simulink model "VirtualMotoTemplate"  (R2025b)
settings: Solver=daessc  StartTime=0  StopTime=2474  FixedStep=.001  RelTol=1e-2  EnableMultiTasking=on
StopFcn:
  | %toc
undefined symbols (not defined in the file): AccelOvrCmd, CtrlTcuInitGear, DecelOvrCmd, Disabled, DriverPreviewDist, EnblAccelOvr, EnblDecelCmd, EnblSteerCmd, EnvAbsPrs, EnvAirTemp, EnvGrvty, EnvNomFrictionScaling, EnvNominalGrade, EnvWindVelX, EnvWindVelY, EnvWindVelZ, FTP75, MotoFrmInert, MotoFrmLngth, MotoFrmMass, MotoLowrFrntFrkMass, MotoRearArmLngth, MotoRearArmMass, MotoUpprFrntFrkMass, RiderLkAhdPtDstGain, RiderMass, ScnAccTbl, ScnBrkTbl, ScnCRMaxLatAccel, ScnCRRadius, ScnDLCGateLongPos, ScnDLCLatRef, ScnDLCLatRefOffset, ScnDLCLongRefBpt, ScnDLCLongRefStartPos, ScnDLCVehicleWidth, ScnFHCounterDwellTime, ScnFHInitialDwellTime, ScnFHReturnTime, ScnFHRollRateZeroCross, ScnFHSteerAmp, ScnFHSteerSpeed, ScnISHandwheelRate, ScnISMaxHandwheelAng, ScnISMaxLatAccel, ScnISSteerHoldTime, ScnLongPosBpts, ScnLongVelRef, ScnOvalTrackl, ScnOvalTrackpdst, ScnOvalTrackr, ScnSDDwellTime, ScnSDSteerAmp, ScnSDSteerFreq, ScnSSFinalFreq, ScnSSSteerAmp, ScnSSSweepTime, ScnStartTime, ScnStrgAngTbl, ScnStrgTrqTbl ... (+10)
libraries: simulink x16, vehdynlibscenariocommon x9, sm_lib x6, autolibshared x4, nesl_utility x4, vehdynlibviscommon x3, sim3dgroundtruthsensorlib x2, vehdynlibdriver x2, sharedtransform x1, autolibutils x1, sim3dautolib x1, sim3dlib x1
(part 5 of 6)

== system VirtualMotoTemplate/Rider Commands/Rider Commands/Roll angle control/Rider Steering Control ==
  sensors : Inport
  TargetRollAngle : Inport  Port=2
  Bus Selector1 : BusSelector  OutputSignals=Wheels.RearTire.Vx,Wheels.RearTire.Gamma,Wheels.RearTire.phidot,Wheels.RearTire.X,Wheels.RearTire.Y,Body.InertFrm.Cg.Ang.psi
  Rider Steering : Subsystem  Variant=on  VariantControlMode=label  VariantControl=Choice  LabelModeActiveChoice=Roll angle control  mask{RiderControlTypePanel=Roll angle control, TrajectoryTypePanel=Oval, RidTrajContG=RidTrajContG, RidTrajContGphi=RidTrajContGphi, RidTrajContGphid=RidTrajContGphid, RidTrajContGl=RidTrajContGl, RidTrajContTD=RidTrajContTD, RidTrajContTL=RidTrajContTL, RidRollContGphi=RidRollContGphi, RidRollContGphid=RidRollContGphid, Trajr=Trajr, Trajl=Trajl, Trajpointdist=Trajpointdist, TrajDatFile=TrajDatFile}
      mask prompts: RiderControlTypePanel "Rider control type:"; TrajectoryTypePanel "Trajectory type:"; RidTrajContG "Gain to determine the Target roll angle, RidContG [rad/m]:"; RidTrajContGphi "Gain to follow the Target trajectory, RidContGphi [Nm/rad]:"; RidTrajContGphid "Gain to prevent the vehicle from tipping over, RidContGphid [Nms/rad]:"; RidTrajContGl "Gain that determines the distance to the look ahead point, RidContGl [s]:"; RidTrajContTD "Time constant for 1st order delay, RidContTD [s]:"; RidTrajContTL "Dead time of rider operation, RidContTL [s]:"; RidRollContGphi "Gain to follow the Target trajectory, RidContGphi [Nm/rad]:"; RidRollContGphid "Gain to prevent the vehicle from tipping over, RidContGphid [Nms/rad]:"; Trajr "Trajectory parameter,Trajr [m]:"; Trajl "Trajectory parameter,Trajl [m]:"; Trajpointdist ",Trajpdist [m]:"; TrajDatFile "Trajectory data file:"
      mask init:
      | maskObj = Simulink.Mask.get(gcb);
      | 
      | Type_tmp = maskObj.getParameter('TrajectoryTypePanel');
      | Type     = Type_tmp.Value;
      | 
      | switch Type
      |     case 'Oval'
      | % ------------------------------------------------------------------------%
      | %  Create Trajectory
      | % ------------------------------------------------------------------------%
      | % --- Oval --- %
      | % top part %
      | x_straight1 = -Trajl/2:Trajpointdist:Trajl/2;
      | y_straight1 = x_straight1*0;
      | 
      | % bottom part %
      | x_straight2 = -Trajl/2:Trajpointdist:Trajl/2;
      | y_straight2 = x_straight1*0+2*Trajr;
      | 
      | % right part %
      | theta_corner1 = -pi/2:Trajpointdist/Trajr:pi/2;
      | x_corner1     = Trajr*cos(theta_corner1)+Trajl/2;
      | y_corner1     = Trajr*sin(theta_corner1)+Trajr;
      | 
      | % left part %
      | theta_corner2 = pi/2:Trajpointdist/Trajr:3/2*pi;
      | x_corner2     = Trajr*cos(theta_corner2)-Trajl/2;
      | y_corner2     = Trajr*sin(theta_corner2)+Trajr;
      | 
      | % total %
      | x_oval = [x_straight1, x_corner1(2:end), fliplr(x_straight2), x_corner2(2:end)];
      | y_oval = [y_straight1, y_corner1(2:end), fliplr(y_straight2), y_corner2(2:end)];
      | 
      | trackData(1,:) = x_oval;
      | trackData(2,:) = y_oval;
      | trackData(3,:) = y_oval*0;
      | 
      |     case 'User defined'
      | 
      | TmpTraj = load(TrajDatFile);
      | 
      | trackData(1,:) = TmpTraj.TrajX;
      | trackData(2,:) = -TmpTraj.TrajY;
      | trackData(3,:) = TmpTraj.TrajY*0;
      | 
      | end
      mask Callback RiderControlTypePanel:
      | maskObj = Simulink.Mask.get(gcb);
      | 
      | Type_tmp = maskObj.getParameter('RiderControlTypePanel');
      | Type     = Type_tmp.Value;
      | 
      | TrajGroup = maskObj.getDialogControl('RiderTrajectoryControlParamPanel');
      | RollGroup = maskObj.getDialogControl('RiderRollControlParamPanel');
      | 
      | TrajectoryTypePanel = maskObj.getDialogControl('TrajectoryTypeCont');
      | TargetTrajectoryParamGroup = maskObj.getDialogControl('TargetTrajectoryParamGroup');
      | 
      | GroupAll = maskObj.getDialogControl('RiderControlParamGroup');
      | 
      | switch Type
      |     case 'None'
      |     set_param(gcb,'LabelModeActiveChoice', 'None');
      |     TrajGroup.Visible = 'off';
      |     RollGroup.Visible = 'off';
      |     GroupAll.Visible  = 'off';
      |     TrajectoryTypePanel.Visible = 'off';
      |     TargetTrajectoryParamGroup.Visible = 'off';
      |     case 'Target trajectory driving - Look ahead point'
      |     set_param(gcb,'LabelModeActiveChoice', 'Target trajectory driving - Look ahead point');
      |     TrajGroup.Visible = 'on';
      |     RollGroup.Visible = 'off';
      |     GroupAll.Visible  = 'on';
      |     TrajectoryTypePanel.Visible = 'on';
      |     TargetTrajectoryParamGroup.Visible = 'on';
      |     case 'Roll angle control'
      |     set_param(gcb,'LabelModeActiveChoice','Roll angle control');
      |     TrajGroup.Visible = 'off';
      |     RollGroup.Visible = 'on';
      |     GroupAll.Visible  = 'on';
      |     TrajectoryTypePanel.Visible = 'off';
      |     TargetTrajectoryParamGroup.Visible = 'off';
      |     case 'External'
      |     set_param(gcb,'LabelModeActiveChoice', 'External');
      |     TrajGroup.Visible = 'off';
      |     RollGroup.Visible = 'off';
      |     GroupAll.Visible  = 'off';
      |     TrajectoryTypePanel.Visible = 'off';
      |     TargetTrajectoryParamGroup.Visible = 'off';
      | end
      mask TypeOptions TrajectoryTypePanel: Oval | User defined
      mask Callback TrajectoryTypePanel:
      | maskObj = Simulink.Mask.get(gcb);
      | 
      | Type_tmp = maskObj.getParameter('TrajectoryTypePanel');
      | Type     = Type_tmp.Value;
      | 
      | TargetTrajectoryParamOvalPanel = maskObj.getDialogControl('TargetTrajectoryParamOvalPanel');
      | 
      | TargetTrajectoryParamUserDefinedPanel = maskObj.getDialogControl('TargetTrajectoryParamUserDefinedPanel');
      | 
      | TargetTrajectoryParamGroup = maskObj.getDialogControl('TargetTrajectoryParamGroup');
      | 
      | switch Type
      |     case 'Oval'
      | TargetTrajectoryParamGroup.Visible = 'on';
      | TargetTrajectoryParamOvalPanel.Visible        = 'on';
      | TargetTrajectoryParamUserDefinedPanel.Visible = 'off';
      |     case 'User defined'
      | TargetTrajectoryParamGroup.Visible = 'on';
      | TargetTrajectoryParamOvalPanel.Visible        = 'off';
      | TargetTrajectoryParamUserDefinedPanel.Visible = 'on';
      | end
      mask DialogControl RiderOptionsGroup Prompt: Options
      mask DialogControl RiderTrajectoryControlParamPanel Prompt: Control parameters
      mask DialogControl RiderRollControlParamPanel Prompt: Control parameters
      mask DialogControl TargetTrajectoryParamOvalPanel Prompt: Trajectory parameters
      mask DialogControl OvalTrajConfBtn Prompt: Confirm
      mask DialogControl OvalTrajConfBtn Callback:
      | maskObj = Simulink.Mask.get(gcb);
      | 
      | Trajr_tmp          = maskObj.getParameter('Trajr');
      | Trajr              = str2num(Trajr_tmp.Value);
      | Trajl_tmp          = maskObj.getParameter('Trajl');
      | Trajl              = str2num(Trajl_tmp.Value);
      | Trajpointdist_tmp  = maskObj.getParameter('Trajpointdist');
      | Trajpointdist      = str2num(Trajpointdist_tmp.Value);
      | 
      | % ------------------------------------------------------------------------%
      | %  Create Trajectory
      | % ------------------------------------------------------------------------%
      | % --- Oval --- %
      | % top part %
      | x_straight1 = -Trajl/2:Trajpointdist:Trajl/2;
      | y_straight1 = x_straight1*0;
      | 
      | % bottom part %
      | x_straight2 = -Trajl/2:Trajpointdist:Trajl/2;
      | y_straight2 = x_straight1*0+2*Trajr;
      | 
      | % right part %
      | theta_corner1 = -pi/2:Trajpointdist/Trajr:pi/2;
      | x_corner1     = Trajr*cos(theta_corner1)+Trajl/2;
      | y_corner1     = Trajr*sin(theta_corner1)+Trajr;
      | 
      | % left part %
      | theta_corner2 = pi/2:Trajpointdist/Trajr:3/2*pi;
      | x_corner2     = Trajr*cos(theta_corner2)-Trajl/2;
      | y_corner2     = Trajr*sin(theta_corner2)+Trajr;
      | 
      | % total %
      | x_oval = [x_straight1, x_corner1(2:end), fliplr(x_straight2), x_corner2(2:end)];
      | y_oval = [y_straight1, y_corner1(2:end), fliplr(y_straight2), y_corner2(2:end)];
      | 
      | figure;
      | plot(x_oval, -y_oval);
      | axis equal;
      | grid on;
      | xlabel('Coordinate X [m]');
      | ylabel('Coordinate Y [m]');
      | title('Oval target trajectory');
      | set(gca,'YDir','reverse')
      mask DialogControl TargetTrajectoryParamUserDefinedPanel Prompt: Trajectory parameters
      mask DialogControl UserDefinedTrajConfBtn Prompt: Confirm
      mask DialogControl UserDefinedTrajConfBtn Callback:
      | maskObj = Simulink.Mask.get(gcb);
      | 
      | File_tmp = maskObj.getParameter('TrajDatFile');
      | File     = replace(File_tmp.Value,'''','');
      | 
      | TmpTraj = load(File);
      | 
      | figure;
      | plot(TmpTraj.TrajX, TmpTraj.TrajY);
      | grid on;
      | xlabel('Coordinate X [m]');
      | ylabel('Coordinate Y [m]');
      | title('User defined target trajectory');
      | set(gca,'YDir','reverse');
  RiderInfo : Outport
  wires:
  sensors/1 -> Bus Selector1/1
  Rider Steering/1(Info) -> RiderInfo/1  "RiderInfo"
  TargetRollAngle/1 -> Rider Steering/7(Target roll angle)
  Bus Selector1/1 -> Rider Steering/1(dxdt)  "<Vx>"
  Bus Selector1/2 -> Rider Steering/2(roll)  "<Gamma>"
  Bus Selector1/3 -> Rider Steering/3(rollRate)  "<phidot>"
  Bus Selector1/4 -> Rider Steering/4(X)  "<X>"
  Bus Selector1/5 -> Rider Steering/5(Y)  "<Y>"
  Bus Selector1/6 -> Rider Steering/6(psi)  "<psi>"

== system VirtualMotoTemplate/Environment/Friction/Varying Friction/Road Track Friction/2D Lookup Tbl for Scaling Fctr (Lambda) ==
  XWhl : Inport  Partition=on  PartitionDimension=1  PartitionWidth=1  PartitionOffset=0
  YWhl : Inport  Port=2  Partition=on  PartitionDimension=1  PartitionWidth=1  PartitionOffset=0
  XBpt : Inport  Port=3
  YBpt : Inport  Port=4
  2-D Lookup Table : Lookup_n-D  BreakpointsForDimension1Source=Input port  BreakpointsForDimension1=xbr  BreakpointsForDimension2Source=Input port  BreakpointsForDimension2=ybr  Table=mutable  ExtrapMethod=Clip  InternalRulePriority=Speed  RndMeth=Simplest
      settings: InputPortMap=u0,u1,p5,p7
  For Each : ForEach  DisableCoverage=on
  Lambda for each whl : Outport  ConcatenationDimension=1
  wires:
  XWhl/1 -> 2-D Lookup Table/1
  YWhl/1 -> 2-D Lookup Table/2
  2-D Lookup Table/1 -> Lambda for each whl/1
  XBpt/1 -> 2-D Lookup Table/3
  YBpt/1 -> 2-D Lookup Table/4

== system VirtualMotoTemplate/Environment/Friction/Varying Friction/Road Track Friction/Creating Inertial Frm Bpt ==
  XCg : Inport
  YCg : Inport  Port=2
  Enable : EnablePort
  Add : Sum
  Add1 : Sum
  Constant1 : Constant  Value=ybr
  Constant3 : Constant  Value=xbr
  XBpt : Outport
  YBpt : Outport  Port=2
  wires:
  Add/1 -> XBpt/1
  Constant1/1 -> Add1/1
  Add1/1 -> YBpt/1
  Constant3/1 -> Add/2
  YCg/1 -> Add1/2
  XCg/1 -> Add/1

== system VirtualMotoTemplate/Environment/Friction/Varying Friction/Road Track Friction/En at t = 0 ==
  Clock1 : Clock
  Compare To Zero : simulink/Logic and Bit Operations/Compare To Zero  relop===  OutDataTypeStr=boolean
  Constant : Constant
  Constant2 : Constant  Value=0
  Switch1 : Switch  Criteria=u2 > Threshold  SaturateOnIntegerOverflow=off  InputSameDT=off
  Out1 : Outport
  wires:
  Clock1/1 -> Compare To Zero/1
  Constant2/1 -> Switch1/3
  Constant/1 -> Switch1/1
  Switch1/1 -> Out1/1
  Compare To Zero/1 -> Switch1/2

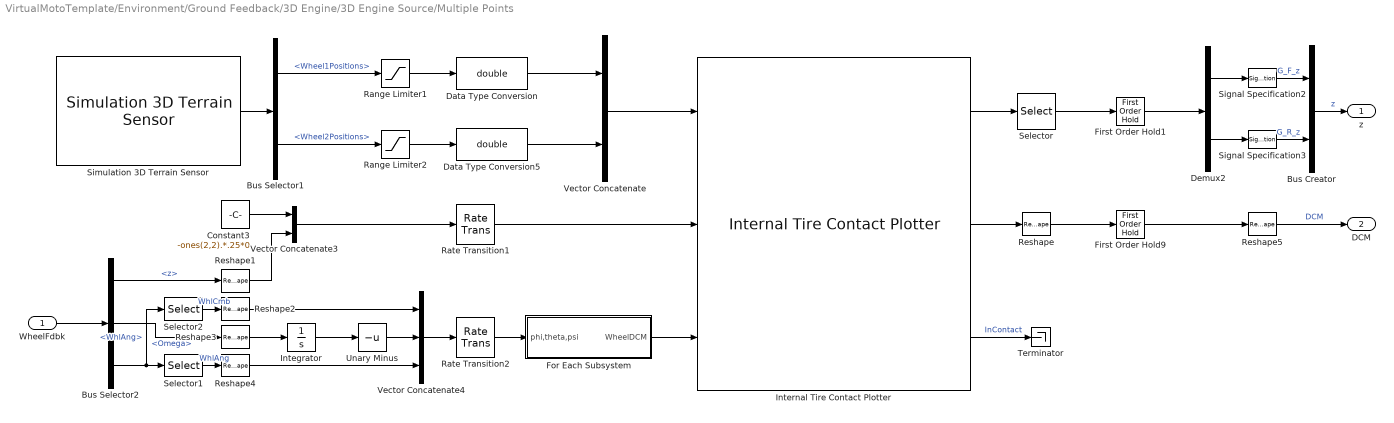
== system VirtualMotoTemplate/Environment/Ground Feedback/3D Engine/3D Engine Source/Multiple Points ==
  WheelFdbk : Inport
  Bus Creator : BusCreator  Inputs=2
  Bus Selector1 : BusSelector  OutputSignals=Wheel1Positions,Wheel2Positions
  Bus Selector2 : BusSelector  OutputSignals=z,Omega,WhlAng
  Constant3 : Constant  Value=-ones(2,2).*.25*0
  Data Type Conversion : DataTypeConversion  OutDataTypeStr=double  SaturateOnIntegerOverflow=off  RndMeth=Floor
  Data Type Conversion5 : DataTypeConversion  OutDataTypeStr=double  SaturateOnIntegerOverflow=off  RndMeth=Floor
  Demux2 : Demux  Outputs=2
  First Order Hold1 : FirstOrderHold  OutputAlgorithm=Fast (Minimize Error)  ErrorTolerance=.001
  First Order Hold9 : FirstOrderHold  InitialOutput=reshape(repmat(eye(3),1,1,2),[],1)  OutputAlgorithm=Fast (Minimize Error)  ErrorTolerance=.001
  For Each Subsystem : Subsystem  TreatAsAtomicUnit=on
  Integrator : Integrator  WrapState=on  ZeroCross=off
  Internal Tire Contact Plotter : vehdynlibviscommon/Internal Tire Contact Plotter  dispFig=off  numAxles=2  numWheelsPerAxle=1  wheelRad=.33  wheelWidth=.235  rayOrigins=[0.5 -0.5 0;0.4 -0.5 0;0.3 -0.5 0;0.19999999999999996 -0.5 0;0.099999999999999978 -0.5 0;0 -0.5 0;-0.099999999999999978 -0.5 0;-0.19999999999999996 -0.5 0;-0.3 -0.5 0;-0.4 -0.5 0;-0.5 -0.5 0;0.5 -0.4 0;0.4 -0.4 0;0.3 -0.4 0;0.19999999999999996 -0.4 0;0.099999999999999978 -0.4 0;0 -0.4 0;-0.099999999999999978 -0.4 0;-0.19999999999999996 -0.4 0;-0.3 -0.4 0;-0.4 -0.4 0;-0.5 -0.4 0;0.5 -0.3 0;0.4 -0.3 0;0.3 -0.3 0;0.19999999999999996 -0.3 0;0.099999999999999978 -0.3 0;0 -0.3 0;-0.099999999999999978 -0.3 0;-0.19999999999999996 -0.3 0;-0.3 -0.3 0;-0.4 -0.3 0;-0.5 -0.3 0;0.5 -0.19999999999999996 0;0.4 -0.19999999999999996 0;0.3 -0.19999999999999996 0;0.19999999999999996 -0.19999999999999996 0;0.099999999999999978 -0.19999999999999996 0;0 -0.19999999999999996 0;-0.099999999999999978 -0.19999999999999996 0;-0.19999999999999996 -0.19999999999999996 0;-0.3 -0.19999999999999996 0;-0.4 -0.19999999999999996 0;-0.5 -0.19999999999999996 0;0.5 -0.099999999999999978 0;0.4 -0.099999999999999978 0;0.3 -0.099999999999999978 0;0.19999999999999996 -0.099999999999999978 0;0.099999999999999978 -0.099999999999999978 0;0 -0.099999999999999978 0;-0.099999999999999978 -0.099999999999999978 0;-0.19999999999999996 -0.099999999999999978 0;-0.3 -0.099999999999999978 0;-0.4 -0.099999999999999978 0;-0.5 -0.099999999999999978 0;0.5 0 0;0.4 0 0;0.3 0 0;0.19999999999999996 0 0;0.099999999999999978 0 0;0 0 0;-0.099999999999999978 0 0;-0.19999999999999996 0 0;-0.3 0 0;-0.4 0 0;-0.5 0 0;0.5 0.099999999999999978 0;0.4 0.099999999999999978 0;0.3 0.099999999999999978 0;0.19999999999999996 0.099999999999999978 0;0.099999999999999978 0.099999999999999978 0;0 0.099999999999999978 0;-0.099999999999999978 0.099999999999999978 0;-0.19999999999999996 0.099999999999999978 0;-0.3 0.099999999999999978 0;-0.4 0.099999999999999978 0;-0.5 0.099999999999999978 0;0.5 0.19999999999999996 0;0.4 0.19999999999999996 0;0.3 0.19999999999999996 0;0.19999999999999996 0.19999999999999996 0;0.099999999999999978 0.19999999999999996 0;0 0.19999999999999996 0;-0.099999999999999978 0.19999999999999996 0;-0.19999999999999996 0.19999999999999996 0;-0.3 0.19999999999999996 0;-0.4 0.19999999999999996 0;-0.5 0.19999999999999996 0;0.5 0.3 0;0.4 0.3 0;0.3 0.3 0;0.19999999999999996 0.3 0;0.099999999999999978 0.3 0;0 0.3 0;-0.099999999999999978 0.3 0;-0.19999999999999996 0.3 0;-0.3 0.3 0;-0.4 0.3 0;-0.5 0.3 0;0.5 0.4 0;0.4 0.4 0;0.3 0.4 0;0.19999999999999996 0.4 0;0.099999999999999978 0.4 0;0 0.4 0;-0.099999999999999978 0.4 0;-0.19999999999999996 0.4 0;-0.3 0.4 0;-0.4 0.4 0;-0.5 0.4 0;0.5 0.5 0;0.4 0.5 0;0.3 0.5 0;0.19999999999999996 0.5 0;0.099999999999999978 0.5 0;0 0.5 0;-0.099999999999999978 0.5 0;-0.19999999999999996 0.5 0;-0.3 0.5 0;-0.4 0.5 0;-0.5 0.5 0]
  Range Limiter1 : Saturate  UpperLimit=1e3  LowerLimit=-1e3  ZeroCross=off
  Range Limiter2 : Saturate  UpperLimit=1e3  LowerLimit=-1e3  ZeroCross=off
  Rate Transition1 : RateTransition  Integrity=off  Deterministic=off  OutPortSampleTime=.01
  Rate Transition2 : RateTransition  Integrity=off  Deterministic=off  OutPortSampleTime=.01
  Reshape : Reshape  OutputDimensionality=Column vector (2-D)
  Reshape1 : Reshape  OutputDimensionality=Column vector (2-D)
  Reshape2 : Reshape  OutputDimensionality=Row vector (2-D)
  Reshape3 : Reshape  OutputDimensionality=Row vector (2-D)
  Reshape4 : Reshape  OutputDimensionality=Row vector (2-D)
  Reshape5 : Reshape  OutputDimensionality=Customize  OutputDimensions=[3,3,2]
  Selector : Selector  NumberOfDimensions=2  InputPortWidth=3  IndexOptions=Select all,Index vector (dialog)  Indices=[1 3],3  OutputSizes=1,1
  Selector1 : Selector  NumberOfDimensions=2  InputPortWidth=3  IndexOptions=Index vector (dialog),Select all  Indices=[3],1  OutputSizes=1,1
  Selector2 : Selector  NumberOfDimensions=2  InputPortWidth=3  IndexOptions=Index vector (dialog),Select all  Indices=[1],1  OutputSizes=1,1
  Signal Specification2 : SignalSpecification  Unit=m
  Signal Specification3 : SignalSpecification  Unit=m
  Simulation 3D Terrain Sensor : sim3dgroundtruthsensorlib/Simulation 3D Terrain Sensor  Priority=1  vehTagList={'Scene Origin';'SimulinkVehicle1'}  sensorTag=Sim3dSensor�  sensorId=1  sensorName=Sim3dSensor�  vehTag=SimulinkVehicle1  CoordinateSystem=Default  tmountOffset=[0, 0, 0]  rmountOffset=[0,0,0,]  RayOrigins=[0.5 -0.5 0;0.4 -0.5 0;0.3 -0.5 0;0.19999999999999996 -0.5 0;0.099999999999999978 -0.5 0;0 -0.5 0;-0.099999999999999978 -0.5 0;-0.19999999999999996 -0.5 0;-0.3 -0.5 0;-0.4 -0.5 0;-0.5 -0.5 0;0.5 -0.4 0;0.4 -0.4 0;0.3 -0.4 0;0.19999999999999996 -0.4 0;0.099999999999999978 -0.4 0;0 -0.4 0;-0.099999999999999978 -0.4 0;-0.19999999999999996 -0.4 0;-0.3 -0.4 0;-0.4 -0.4 0;-0.5 -0.4 0;0.5 -0.3 0;0.4 -0.3 0;0.3 -0.3 0;0.19999999999999996 -0.3 0;0.099999999999999978 -0.3 0;0 -0.3 0;-0.099999999999999978 -0.3 0;-0.19999999999999996 -0.3 0;-0.3 -0.3 0;-0.4 -0.3 0;-0.5 -0.3 0;0.5 -0.19999999999999996 0;0.4 -0.19999999999999996 0;0.3 -0.19999999999999996 0;0.19999999999999996 -0.19999999999999996 0;0.099999999999999978 -0.19999999999999996 0;0 -0.19999999999999996 0;-0.099999999999999978 -0.19999999999999996 0;-0.19999999999999996 -0.19999999999999996 0;-0.3 -0.19999999999999996 0;-0.4 -0.19999999999999996 0;-0.5 -0.19999999999999996 0;0.5 -0.099999999999999978 0;0.4 -0.099999999999999978 0;0.3 -0.099999999999999978 0;0.19999999999999996 -0.099999999999999978 0;0.099999999999999978 -0.099999999999999978 0;0 -0.099999999999999978 0;-0.099999999999999978 -0.099999999999999978 0;-0.19999999999999996 -0.099999999999999978 0;-0.3 -0.099999999999999978 0;-0.4 -0.099999999999999978 0;-0.5 -0.099999999999999978 0;0.5 0 0;0.4 0 0;0.3 0 0;0.19999999999999996 0 0;0.099999999999999978 0 0;0 0 0;-0.099999999999999978 0 0;-0.19999999999999996 0 0;-0.3 0 0;-0.4 0 0;-0.5 0 0;0.5 0.099999999999999978 0;0.4 0.099999999999999978 0;0.3 0.099999999999999978 0;0.19999999999999996 0.099999999999999978 0;0.099999999999999978 0.099999999999999978 0;0 0.099999999999999978 0;-0.099999999999999978 0.099999999999999978 0;-0.19999999999999996 0.099999999999999978 0;-0.3 0.099999999999999978 0;-0.4 0.099999999999999978 0;-0.5 0.099999999999999978 0;0.5 0.19999999999999996 0;0.4 0.19999999999999996 0;0.3 0.19999999999999996 0;0.19999999999999996 0.19999999999999996 0;0.099999999999999978 0.19999999999999996 0;0 0.19999999999999996 0;-0.099999999999999978 0.19999999999999996 0;-0.19999999999999996 0.19999999999999996 0;-0.3 0.19999999999999996 0;-0.4 0.19999999999999996 0;-0.5 0.19999999999999996 0;0.5 0.3 0;0.4 0.3 0;0.3 0.3 0;0.19999999999999996 0.3 0;0.099999999999999978 0.3 0;0 0.3 0;-0.099999999999999978 0.3 0;-0.19999999999999996 0.3 0;-0.3 0.3 0;-0.4 0.3 0;-0.5 0.3 0;0.5 0.4 0;0.4 0.4 0;0.3 0.4 0;0.19999999999999996 0.4 0;0.099999999999999978 0.4 0;0 0.4 0;-0.099999999999999978 0.4 0;-0.19999999999999996 0.4 0;-0.3 0.4 0;-0.4 0.4 0;-0.5 0.4 0;0.5 0.5 0;0.4 0.5 0;0.3 0.5 0;0.19999999999999996 0.5 0;0.099999999999999978 0.5 0;0 0.5 0;-0.099999999999999978 0.5 0;-0.19999999999999996 0.5 0;-0.3 0.5 0;-0.4 0.5 0;-0.5 0.5 0]  RayDirections=[0 0 -1;0 0 -1;0 0 -1;0 0 -1;0 0 -1;0 0 -1;0 0 -1;0 0 -1;0 0 -1;0 0 -1;0 0 -1;0 0 -1;0 0 -1;0 0 -1;0 0 -1;0 0 -1;0 0 -1;0 0 -1;0 0 -1;0 0 -1;0 0 -1;0 0 -1;0 0 -1;0 0 -1;0 0 -1;0 0 -1;0 0 -1;0 0 -1;0 0 -1;0 0 -1;0 0 -1;0 0 -1;0 0 -1;0 0 -1;0 0 -1;0 0 -1;0 0 -1;0 0 -1;0 0 -1;0 0 -1;0 0 -1;0 0 -1;0 0 -1;0 0 -1;0 0 -1;0 0 -1;0 0 -1;0 0 -1;0 0 -1;0 0 -1;0 0 -1;0 0 -1;0 0 -1;0 0 -1;0 0 -1;0 0 -1;0 0 -1;0 0 -1;0 0 -1;0 0 -1;0 0 -1;0 0 -1;0 0 -1;0 0 -1;0 0 -1;0 0 -1;0 0 -1;0 0 -1;0 0 -1;0 0 -1;0 0 -1;0 0 -1;0 0 -1;0 0 -1;0 0 -1;0 0 -1;0 0 -1;0 0 -1;0 0 -1;0 0 -1;0 0 -1;0 0 -1;0 0 -1;0 0 -1;0 0 -1;0 0 -1;0 0 -1;0 0 -1;0 0 -1;0 0 -1;0 0 -1;0 0 -1;0 0 -1;0 0 -1;0 0 -1;0 0 -1;0 0 -1;0 0 -1;0 0 -1;0 0 -1;0 0 -1;0 0 -1;0 0 -1;0 0 -1;0 0 -1;0 0 -1;0 0 -1;0 0 -1;0 0 -1;0 0 -1;0 0 -1;0 0 -1;0 0 -1;0 0 -1;0 0 -1;0 0 -1;0 0 -1;0 0 -1;0 0 -1;0 0 -1;0 0 -1]  RayLengths=[20;20;20;20;20;20;20;20;20;20;20;20;20;20;20;20;20;20;20;20;20;20;20;20;20;20;20;20;20;20;20;20;20;20;20;20;20;20;20;20;20;20;20;20;20;20;20;20;20;20;20;20;20;20;20;20;20;20;20;20;20;20;20;20;20;20;20;20;20;20;20;20;20;20;20;20;20;20;20;20;20;20;20;20;20;20;20;20;20;20;20;20;20;20;20;20;20;20;20;20;20;20;20;20;20;20;20;20;20;20;20;20;20;20;20;20;20;20;20;20;20]  NumberOfWheels=2  VisualizeTraceLines=off  SampleTime=-1  aMode=2  ID=1
  Terminator : Terminator
  Unary Minus : UnaryMinus
  Vector Concatenate : Concatenate  Mode=Multidimensional array  ConcatenateDimension=3
  Vector Concatenate3 : Concatenate  Mode=Multidimensional array  ConcatenateDimension=2
  Vector Concatenate4 : Concatenate  NumInputs=3  Mode=Multidimensional array
  z : Outport
  DCM : Outport  Port=2
  wires:
  Selector2/1 -> Reshape2/1  "WhlCmb"
  Selector1/1 -> Reshape4/1  "WhlAng"
  First Order Hold1/1 -> Demux2/1
  Reshape/1 -> First Order Hold9/1
  First Order Hold9/1 -> Reshape5/1
  Rate Transition1/1 -> Internal Tire Contact Plotter/2
  Unary Minus/1 -> Vector Concatenate4/2
  Reshape2/1 -> Vector Concatenate4/1
  Constant3/1 -> Vector Concatenate3/1
  Bus Selector2/3 -> Selector1/1, Selector2/1  "<WhlAng>"
  Bus Selector2/1 -> Reshape1/1  "<z>"
  WheelFdbk/1 -> Bus Selector2/1
  Reshape1/1 -> Vector Concatenate3/2
  Rate Transition2/1 -> For Each Subsystem/1(phi,theta,psi)
  Reshape4/1 -> Vector Concatenate4/3
  Vector Concatenate4/1 -> Rate Transition2/1
  Reshape3/1 -> Integrator/1
  For Each Subsystem/1(WheelDCM) -> Internal Tire Contact Plotter/3
  Vector Concatenate3/1 -> Rate Transition1/1
  Bus Selector2/2 -> Reshape3/1  "<Omega>"
  Integrator/1 -> Unary Minus/1
  Internal Tire Contact Plotter/2 -> Reshape/1
  Reshape5/1 -> DCM/1  "DCM"
  Range Limiter1/1 -> Data Type Conversion/1
  Simulation 3D Terrain Sensor/1 -> Bus Selector1/1
  Demux2/1 -> Signal Specification2/1
  Bus Selector1/2 -> Range Limiter2/1  "<Wheel2Positions>"
  Signal Specification3/1 -> Bus Creator/2  "G_R_z"
  Signal Specification2/1 -> Bus Creator/1  "G_F_z"
  Bus Creator/1 -> z/1  "z"
  Bus Selector1/1 -> Range Limiter1/1  "<Wheel1Positions>"
  Vector Concatenate/1 -> Internal Tire Contact Plotter/1
  Internal Tire Contact Plotter/3 -> Terminator/1  "InContact"
  Internal Tire Contact Plotter/1 -> Selector/1
  Data Type Conversion5/1 -> Vector Concatenate/2
  Data Type Conversion/1 -> Vector Concatenate/1
  Demux2/2 -> Signal Specification3/1
  Selector/1 -> First Order Hold1/1
  Range Limiter2/1 -> Data Type Conversion5/1

== system VirtualMotoTemplate/Environment/Ground Feedback/3D Engine/3D Engine Source/Single Point ==
  Bus Creator1 : BusCreator  Inputs=2
  Bus Selector2 : BusSelector  OutputSignals=Wheel1Positions,Wheel2Positions
  Constant2 : Constant  Value=repmat(eye(3),1,1,2)  SampleTime=-1
  Data Type Conversion1 : DataTypeConversion  SaturateOnIntegerOverflow=off  RndMeth=Floor
  Data Type Conversion2 : DataTypeConversion  SaturateOnIntegerOverflow=off  RndMeth=Floor
  First Order Hold5 : FirstOrderHold  ErrorTolerance=1
  First Order Hold6 : FirstOrderHold  ErrorTolerance=1
  Range Limiter5 : Saturate  UpperLimit=1e3  LowerLimit=-1e3  ZeroCross=off
  Range Limiter6 : Saturate  UpperLimit=1e3  LowerLimit=-1e3  ZeroCross=off
  Signal Specification6 : SignalSpecification  Unit=m
  Signal Specification7 : SignalSpecification  Unit=m
  Simulation 3D Terrain Sensor1 : sim3dgroundtruthsensorlib/Simulation 3D Terrain Sensor  Priority=1  vehTagList={'Scene Origin';'SimulinkVehicle1'}  sensorTag=Sim3dSensor�  sensorId=1  sensorName=Sim3dSensor�  vehTag=SimulinkVehicle1  CoordinateSystem=Default  tmountOffset=[0, 0, 0]  rmountOffset=[0,0,0,]  RayOrigins=[0 0 1]  RayDirections=[0 0 -1]  RayLengths=20  NumberOfWheels=2  VisualizeTraceLines=off  SampleTime=-1  aMode=2  ID=1
  Zend Select1 : Selector  NumberOfDimensions=2  InputPortWidth=3  IndexOptions=Select all,Index vector (dialog)  Indices=[1 3],3  OutputSizes=1,1
  Zend Select2 : Selector  NumberOfDimensions=2  InputPortWidth=3  IndexOptions=Select all,Index vector (dialog)  Indices=[1 3],3  OutputSizes=1,1
  z : Outport
  DCM : Outport  Port=2
  wires:
  Constant2/1 -> DCM/1  "DCM"
  Bus Creator1/1 -> z/1  "z"
  Range Limiter5/1 -> Zend Select1/1
  First Order Hold5/1 -> Signal Specification6/1
  Bus Selector2/1 -> Range Limiter5/1  "<Wheel1Positions>"
  Data Type Conversion1/1 -> First Order Hold5/1
  Range Limiter6/1 -> Zend Select2/1
  Data Type Conversion2/1 -> First Order Hold6/1
  Zend Select2/1 -> Data Type Conversion2/1
  First Order Hold6/1 -> Signal Specification7/1
  Bus Selector2/2 -> Range Limiter6/1  "<Wheel2Positions>"
  Signal Specification7/1 -> Bus Creator1/2  "G_R_z"
  Zend Select1/1 -> Data Type Conversion1/1
  Simulation 3D Terrain Sensor1/1 -> Bus Selector2/1
  Signal Specification6/1 -> Bus Creator1/1  "G_F_z"

== system VirtualMotoTemplate/Reference Generator for Motorcycle/Reference Router/Steering Command Override/Control Signals/Position-Based Angle ==
  Time : Inport
  Position : Inport  Port=2
  1-D Lookup Table : Lookup_n-D  NumberOfTableDimensions=1  BreakpointsForDimension1=LongPosBpts  Table=StrgAngTbl  InternalRulePriority=Speed  RndMeth=Simplest
  Terminator : Terminator
  Steer : Outport
  wires:
  1-D Lookup Table/1 -> Steer/1
  Time/1 -> Terminator/1
  Position/1 -> 1-D Lookup Table/1

== system VirtualMotoTemplate/Reference Generator for Motorcycle/Reference Router/Steering Command Override/Control Signals/Position-Based Torque ==
  Time : Inport
  Position : Inport  Port=2
  1-D Lookup Table : Lookup_n-D  NumberOfTableDimensions=1  BreakpointsForDimension1=LongPosBpts  Table=StrgTrqTbl  InternalRulePriority=Speed  RndMeth=Simplest
  Terminator : Terminator
  Steer : Outport
  wires:
  1-D Lookup Table/1 -> Steer/1
  Position/1 -> 1-D Lookup Table/1
  Time/1 -> Terminator/1

== system VirtualMotoTemplate/Reference Generator for Motorcycle/Reference Router/Steering Command Override/Control Signals/Time-Based Angle ==
  Time : Inport
  Position : Inport  Port=2
  1-D Lookup Table : Lookup_n-D  NumberOfTableDimensions=1  BreakpointsForDimension1=ScnTimeBpts  Table=StrgAngTbl  InternalRulePriority=Speed  RndMeth=Simplest
  Terminator : Terminator
  Steer : Outport
  wires:
  1-D Lookup Table/1 -> Steer/1
  Time/1 -> 1-D Lookup Table/1
  Position/1 -> Terminator/1

== system VirtualMotoTemplate/Reference Generator for Motorcycle/Reference Router/Steering Command Override/Control Signals/Time-Based Torque ==
  Time : Inport
  Position : Inport  Port=2
  1-D Lookup Table : Lookup_n-D  NumberOfTableDimensions=1  BreakpointsForDimension1=TimeBpts  Table=StrgTrqTbl  InternalRulePriority=Speed  RndMeth=Simplest
  Terminator : Terminator
  Steer : Outport
  wires:
  1-D Lookup Table/1 -> Steer/1
  Time/1 -> 1-D Lookup Table/1
  Position/1 -> Terminator/1

== system VirtualMotoTemplate/Reference Generator for Motorcycle/Reference Router/Steering and Accel and Brk Command Override/Control Signals/Position-Based Angle ==
  Time : Inport
  Position : Inport  Port=2
  1-D Lookup Table : Lookup_n-D  NumberOfTableDimensions=1  BreakpointsForDimension1=LongPosBpts  Table=StrgAngTbl  InternalRulePriority=Speed  RndMeth=Simplest
  1-D Lookup Table1 : Lookup_n-D  NumberOfTableDimensions=1  BreakpointsForDimension1=ScnLongPosBpts  Table=AccTbl  InternalRulePriority=Speed  RndMeth=Simplest
  1-D Lookup Table2 : Lookup_n-D  NumberOfTableDimensions=1  BreakpointsForDimension1=LongPosBpts  Table=BrkTbl  InternalRulePriority=Speed  RndMeth=Simplest
  Terminator : Terminator
  Steer : Outport
  Accel : Outport  Port=2
  Brake : Outport  Port=3
  wires:
  1-D Lookup Table/1 -> Steer/1
  1-D Lookup Table1/1 -> Accel/1
  Time/1 -> Terminator/1
  1-D Lookup Table2/1 -> Brake/1
  Position/1 -> 1-D Lookup Table2/1, 1-D Lookup Table1/1, 1-D Lookup Table/1

== system VirtualMotoTemplate/Reference Generator for Motorcycle/Reference Router/Steering and Accel and Brk Command Override/Control Signals/Position-Based Torque ==
  Time : Inport
  Position : Inport  Port=2
  1-D Lookup Table : Lookup_n-D  NumberOfTableDimensions=1  BreakpointsForDimension1=LongPosBpts  Table=StrgTrqTbl  InternalRulePriority=Speed  RndMeth=Simplest
  1-D Lookup Table1 : Lookup_n-D  NumberOfTableDimensions=1  BreakpointsForDimension1=LongPosBpts  Table=AccTbl  InternalRulePriority=Speed  RndMeth=Simplest
  1-D Lookup Table2 : Lookup_n-D  NumberOfTableDimensions=1  BreakpointsForDimension1=LongPosBpts  Table=BrkTbl  InternalRulePriority=Speed  RndMeth=Simplest
  Terminator : Terminator
  Steer : Outport
  Accel : Outport  Port=2
  Brake : Outport  Port=3
  wires:
  1-D Lookup Table/1 -> Steer/1
  Position/1 -> 1-D Lookup Table2/1, 1-D Lookup Table1/1, 1-D Lookup Table/1
  1-D Lookup Table1/1 -> Accel/1
  1-D Lookup Table2/1 -> Brake/1
  Time/1 -> Terminator/1

== system VirtualMotoTemplate/Reference Generator for Motorcycle/Reference Router/Steering and Accel and Brk Command Override/Control Signals/Time-Based Angle ==
  Time : Inport
  Position : Inport  Port=2
  1-D Lookup Table : Lookup_n-D  NumberOfTableDimensions=1  BreakpointsForDimension1=ScnTimeBpts  Table=StrgAngTbl  InternalRulePriority=Speed  RndMeth=Simplest
  1-D Lookup Table1 : Lookup_n-D  NumberOfTableDimensions=1  BreakpointsForDimension1=TimeBpts  Table=AccTbl  InternalRulePriority=Speed  RndMeth=Simplest
  1-D Lookup Table2 : Lookup_n-D  NumberOfTableDimensions=1  BreakpointsForDimension1=ScnTimeBpts  Table=BrkTbl  InternalRulePriority=Speed  RndMeth=Simplest
  Terminator : Terminator
  Steer : Outport
  Accel : Outport  Port=2
  Brake : Outport  Port=3
  wires:
  1-D Lookup Table/1 -> Steer/1
  1-D Lookup Table1/1 -> Accel/1
  1-D Lookup Table2/1 -> Brake/1
  Time/1 -> 1-D Lookup Table2/1, 1-D Lookup Table1/1, 1-D Lookup Table/1
  Position/1 -> Terminator/1

== system VirtualMotoTemplate/Reference Generator for Motorcycle/Reference Router/Steering and Accel and Brk Command Override/Control Signals/Time-Based Torque ==
  Time : Inport
  Position : Inport  Port=2
  1-D Lookup Table : Lookup_n-D  NumberOfTableDimensions=1  BreakpointsForDimension1=TimeBpts  Table=StrgTrqTbl  InternalRulePriority=Speed  RndMeth=Simplest
  1-D Lookup Table1 : Lookup_n-D  NumberOfTableDimensions=1  BreakpointsForDimension1=TimeBpts  Table=AccTbl  InternalRulePriority=Speed  RndMeth=Simplest
  1-D Lookup Table2 : Lookup_n-D  NumberOfTableDimensions=1  BreakpointsForDimension1=TimeBpts  Table=BrkTbl  InternalRulePriority=Speed  RndMeth=Simplest
  Terminator : Terminator
  Steer : Outport
  Accel : Outport  Port=2
  Brake : Outport  Port=3
  wires:
  1-D Lookup Table/1 -> Steer/1
  1-D Lookup Table1/1 -> Accel/1
  1-D Lookup Table2/1 -> Brake/1
  Time/1 -> 1-D Lookup Table2/1, 1-D Lookup Table1/1, 1-D Lookup Table/1
  Position/1 -> Terminator/1

== system VirtualMotoTemplate/Rider Commands/Rider Commands/Longitudinal Rider/Hill Hold/Igore Initialization Transients (t<=2s) ==
  <xdot> : Inport
  Clock : Clock
  Dead Zone : DeadZone  ZeroCross=off
  Switch2 : Switch  Threshold=2  ZeroCross=off  SaturateOnIntegerOverflow=off  InputSameDT=off
  VelFdbk : Outport
  wires:
  Dead Zone/1 -> Switch2/3
  Clock/1 -> Switch2/2
  <xdot>/1 -> Dead Zone/1, Switch2/1
  Switch2/1 -> VelFdbk/1

== system VirtualMotoTemplate/Rider Commands/Rider Commands/Predictive Rider/Hill Hold/Igore Initialization Transients (t<=2s) ==
  <xdot> : Inport
  Clock : Clock
  Dead Zone : DeadZone  ZeroCross=off
  Switch2 : Switch  Threshold=2  ZeroCross=off  SaturateOnIntegerOverflow=off  InputSameDT=off
  VelFdbk : Outport
  wires:
  Dead Zone/1 -> Switch2/3
  Clock/1 -> Switch2/2
  <xdot>/1 -> Dead Zone/1, Switch2/1
  Switch2/1 -> VelFdbk/1

== system VirtualMotoTemplate/Rider Commands/Rider Commands/Predictive Stanley Rider/Hill Hold/Igore Initialization Transients (t<=2s) ==
  <xdot> : Inport
  Clock : Clock
  Dead Zone : DeadZone  ZeroCross=off
  Switch2 : Switch  Threshold=2  ZeroCross=off  SaturateOnIntegerOverflow=off  InputSameDT=off
  VelFdbk : Outport
  wires:
  Dead Zone/1 -> Switch2/3
  Clock/1 -> Switch2/2
  <xdot>/1 -> Dead Zone/1, Switch2/1
  Switch2/1 -> VelFdbk/1

== system VirtualMotoTemplate/Rider Commands/Rider Commands/Roll angle control/Rider Steering Control/Rider Steering ==
  dxdt : Inport
  roll : Inport  Port=2
  rollRate : Inport  Port=3
  X : Inport  Port=4
  Y : Inport  Port=5
  psi : Inport  Port=6
  Target roll angle : Inport  Port=7
  External : Subsystem  VariantControl=External
  None : Subsystem  VariantControl=None
  Roll angle control : Subsystem  VariantControl=Roll angle control
  Target trajectory driving - Look ahead point : Subsystem  VariantControl=Target trajectory driving - Look ahead point
  Info : Outport

== system VirtualMotoTemplate/Environment/Ground Feedback/3D Engine/3D Engine Source/Multiple Points/For Each Subsystem ==
  phi,theta,psi : Inport  Partition=on  PartitionDimension=2  PartitionWidth=1  PartitionOffset=0
  For Each : ForEach  DisableCoverage=on
  Rotation Angles to Direction Cosine Matrix1 : sharedtransform/Rotation Angles to Direction Cosine Matrix  rotationOrder=YXZ  aMode=2
  Selector5 : Selector  InputPortWidth=3  IndexOptions=Index vector (dialog)  Indices=[2 1 3]  OutputSizes=1
  WheelDCM : Outport  ConcatenationDimension=3
  wires:
  phi,theta,psi/1 -> Selector5/1
  Rotation Angles to Direction Cosine Matrix1/1 -> WheelDCM/1
  Selector5/1 -> Rotation Angles to Direction Cosine Matrix1/1

== system VirtualMotoTemplate/Rider Commands/Rider Commands/Roll angle control/Rider Steering Control/Rider Steering/External ==
  Bus Creator : BusCreator  Inputs=3
  Bus Creator1 : BusCreator  Inputs=2
  Ground : Ground
  NaN : Constant  Value=NaN  OutDataTypeStr=Inherit: Inherit via back propagation
  NaN1 : Constant  Value=NaN  OutDataTypeStr=Inherit: Inherit via back propagation
  NaN2 : Constant  Value=NaN  OutDataTypeStr=Inherit: Inherit via back propagation
  Info : Outport
  wires:
  Ground/1 -> Bus Creator/1  "MSteer"
  Bus Creator1/1 -> Bus Creator/2  "LAP"
  Bus Creator/1 -> Info/1  "RiderInfo"
  NaN1/1 -> Bus Creator/3  "mindist"
  NaN2/1 -> Bus Creator1/2  "Y"
  NaN/1 -> Bus Creator1/1  "X"

== system VirtualMotoTemplate/Rider Commands/Rider Commands/Roll angle control/Rider Steering Control/Rider Steering/None ==
  Bus Creator : BusCreator  Inputs=3
  Bus Creator1 : BusCreator  Inputs=2
  Ground : Ground
  NaN1 : Constant  Value=NaN  OutDataTypeStr=Inherit: Inherit via back propagation
  NaN2 : Constant  Value=NaN  OutDataTypeStr=Inherit: Inherit via back propagation
  NaN3 : Constant  Value=NaN  OutDataTypeStr=Inherit: Inherit via back propagation
  Info : Outport
  wires:
  Bus Creator/1 -> Info/1  "RiderInfo"
  Bus Creator1/1 -> Bus Creator/2  "LAP"
  Ground/1 -> Bus Creator/1  "MSteer"
  NaN1/1 -> Bus Creator/3  "mindist"
  NaN2/1 -> Bus Creator1/1  "X"
  NaN3/1 -> Bus Creator1/2  "Y"

== system VirtualMotoTemplate/Rider Commands/Rider Commands/Roll angle control/Rider Steering Control/Rider Steering/Roll angle control ==
  Target roll angle : Inport
  roll : Inport  Port=2
  rollRate : Inport  Port=3
  Add10 : Sum  Inputs=|+-
  Add11 : Sum
  Bus Creator : BusCreator  Inputs=3
  Bus Creator1 : BusCreator  Inputs=2
  Gain24 : Gain  Gain=RidRollContGphid
  Gain27 : Gain  Gain=RidRollContGphi
  NaN : Constant  Value=NaN  OutDataTypeStr=Inherit: Inherit via back propagation
  NaN1 : Constant  Value=NaN  OutDataTypeStr=Inherit: Inherit via back propagation
  NaN2 : Constant  Value=NaN  OutDataTypeStr=Inherit: Inherit via back propagation
  Info : Outport
  wires:
  Add10/1 -> Gain27/1
  Gain27/1 -> Add11/1
  Target roll angle/1 -> Add10/1
  Gain24/1 -> Add11/2
  roll/1 -> Add10/2
  rollRate/1 -> Gain24/1
  Bus Creator/1 -> Info/1  "RiderInfo"
  Bus Creator1/1 -> Bus Creator/2  "LAP"
  Add11/1 -> Bus Creator/1  "MSteer"
  NaN/1 -> Bus Creator1/1  "X"
  NaN1/1 -> Bus Creator/3  "mindist"
  NaN2/1 -> Bus Creator1/2  "Y"

== system VirtualMotoTemplate/Rider Commands/Rider Commands/Roll angle control/Rider Steering Control/Rider Steering/Target trajectory driving - Look ahead point ==
  roll : Inport
  rollRate : Inport  Port=2
  dxdt : Inport  Port=3
  psi : Inport  Port=4
  X : Inport  Port=5
  Y : Inport  Port=6
  Bus Creator : BusCreator  Inputs=3
  Bus Creator1 : BusCreator  Inputs=2
  First Order Hold1 : FirstOrderHold  ErrorTolerance=inf
  LAP calc. : Subsystem
  LAPview : Subsystem
  LateralDeviationDeriver : MATLAB Function  TreatAsAtomicUnit=on
  Transfer Fcn : TransferFcn  Denominator=[RidTrajContTD 1]
  Transport Delay : TransportDelay  DelayTime=RidTrajContTL
  feedback : Subsystem
  Info : Outport
  wires:
  First Order Hold1/1 -> feedback/1(mindist)
  LAP calc./1(x) -> LateralDeviationDeriver/1(current_x), Bus Creator1/1, LAPview/1(px)  "X"
  rollRate/1 -> feedback/3(rollRate)
  feedback/1(control torque) -> Transfer Fcn/1
  Transfer Fcn/1 -> Transport Delay/1
  LateralDeviationDeriver/1(mindist_out) -> Bus Creator/3, First Order Hold1/1  "mindist"
  Y/1 -> LAP calc./4(Y)
  LAP calc./2(y) -> LateralDeviationDeriver/2(current_y), Bus Creator1/2, LAPview/2(pz)  "Y"
  LAP calc./3(-psi) -> LateralDeviationDeriver/3(VehicleYaw)
  Bus Creator1/1 -> Bus Creator/2  "LAP"
  roll/1 -> feedback/2(roll)
  psi/1 -> LAP calc./2(psi)
  X/1 -> LAP calc./3(X)
  dxdt/1 -> LAP calc./1(dxdt)
  Transport Delay/1 -> Bus Creator/1  "MSteer"
  Bus Creator/1 -> Info/1  "RiderInfo"

== system VirtualMotoTemplate/Rider Commands/Rider Commands/Roll angle control/Rider Steering Control/Rider Steering/Target trajectory driving - Look ahead point/LAP calc. ==
  dxdt : Inport
  psi : Inport  Port=2
  X : Inport  Port=3
  Y : Inport  Port=4
  Add : Sum
  Add1 : Sum
  Gain2 : Gain  Gain=RidTrajContGl
  Product : Product
  Product1 : Product
  Trigonometric Function : Trigonometry  Operator=cos
  Trigonometric Function1 : Trigonometry
  Unary Minus : UnaryMinus
  Unary Minus1 : UnaryMinus
  x : Outport
  y : Outport  Port=2
  -psi : Outport  Port=3
  wires:
  Trigonometric Function/1 -> Product/2
  Unary Minus/1 -> -psi/1, Trigonometric Function1/1, Trigonometric Function/1
  Unary Minus1/1 -> Add1/2
  Gain2/1 -> Product1/1, Product/1  "Look ahead point [m]"
  Add1/1 -> y/1
  Product1/1 -> Add1/1
  Y/1 -> Unary Minus1/1
  Product/1 -> Add/1
  Trigonometric Function1/1 -> Product1/2
  dxdt/1 -> Gain2/1
  X/1 -> Add/2
  Add/1 -> x/1
  psi/1 -> Unary Minus/1

== system VirtualMotoTemplate/Rider Commands/Rider Commands/Roll angle control/Rider Steering Control/Rider Steering/Target trajectory driving - Look ahead point/LAPview ==
  px : Inport
  pz : Inport  Port=2
  Cartesian Joint : sm_lib/Joints/Cartesian Joint  JointMode=Normal  CompositeWrenchDir=FollowerOnBase  CompositeWrenchFrame=BaseFrame  SenseConstraintForce=off  SenseConstraintTorque=off  SenseTotalForce=off  SenseTotalTorque=off  PxPositionTargetSpecify=on  PxPositionTargetPriority=High  PxPositionTargetValue=5  PxPositionTargetValueUnits=m  PxVelocityTargetSpecify=off  PxVelocityTargetPriority=High  PxVelocityTargetValue=0  PxVelocityTargetValueUnits=m/s  PxEquilibriumPosition=0  PxEquilibriumPositionUnits=m  PxSpringStiffness=0  PxSpringStiffnessUnits=N/m  PxDampingCoefficient=0  PxDampingCoefficientUnits=N/(m/s)  PxLowerLimitSpecify=off  PxLowerLimitBound=-1  PxLowerLimitBoundUnits=m  PxLowerLimitStiffness=1e6  PxLowerLimitStiffnessUnits=N/m  PxLowerLimitDamping=1e3  PxLowerLimitDampingUnits=N/(m/s)  PxLowerLimitTransitionRegionWidth=1e-4  PxLowerLimitTransitionRegionWidthUnits=m  PxUpperLimitSpecify=off  PxUpperLimitBound=1  PxUpperLimitBoundUnits=m  PxUpperLimitStiffness=1e6  PxUpperLimitStiffnessUnits=N/m  PxUpperLimitDamping=1e3  PxUpperLimitDampingUnits=N/(m/s)  PxUpperLimitTransitionRegionWidth=1e-4  PxUpperLimitTransitionRegionWidthUnits=m  PxTorqueActuationMode=ComputedTorque  PxMotionActuationMode=InputMotion  PxSensePosition=off  PxSenseVelocity=off  PxSenseAcceleration=off  PxSenseTorqueForce=off  PxSenseLowerLimitTorqueForce=off  PxSenseUpperLimitTorqueForce=off  PyPositionTargetSpecify=off  PyPositionTargetPriority=High  PyPositionTargetValue=0  PyPositionTargetValueUnits=m  PyVelocityTargetSpecify=off  PyVelocityTargetPriority=High  PyVelocityTargetValue=0  PyVelocityTargetValueUnits=m/s  PyEquilibriumPosition=0  PyEquilibriumPositionUnits=m  PySpringStiffness=0  PySpringStiffnessUnits=N/m  PyDampingCoefficient=0  PyDampingCoefficientUnits=N/(m/s)  PyLowerLimitSpecify=off  PyLowerLimitBound=-1  PyLowerLimitBoundUnits=m  PyLowerLimitStiffness=1e6  PyLowerLimitStiffnessUnits=N/m  PyLowerLimitDamping=1e3  PyLowerLimitDampingUnits=N/(m/s)  PyLowerLimitTransitionRegionWidth=1e-4  PyLowerLimitTransitionRegionWidthUnits=m  PyUpperLimitSpecify=off  PyUpperLimitBound=1  PyUpperLimitBoundUnits=m  PyUpperLimitStiffness=1e6  PyUpperLimitStiffnessUnits=N/m  PyUpperLimitDamping=1e3  PyUpperLimitDampingUnits=N/(m/s)  PyUpperLimitTransitionRegionWidth=1e-4  PyUpperLimitTransitionRegionWidthUnits=m  PyTorqueActuationMode=ComputedTorque  PyMotionActuationMode=InputMotion  PySensePosition=off  PySenseVelocity=off  PySenseAcceleration=off  PySenseTorqueForce=off  PySenseLowerLimitTorqueForce=off  PySenseUpperLimitTorqueForce=off  PzPositionTargetSpecify=off  PzPositionTargetPriority=High  PzPositionTargetValue=0  PzPositionTargetValueUnits=m  PzVelocityTargetSpecify=off  PzVelocityTargetPriority=High  PzVelocityTargetValue=0  PzVelocityTargetValueUnits=m/s  PzEquilibriumPosition=0  PzEquilibriumPositionUnits=m  PzSpringStiffness=0  PzSpringStiffnessUnits=N/m  PzDampingCoefficient=0  PzDampingCoefficientUnits=N/(m/s)  PzLowerLimitSpecify=off  PzLowerLimitBound=-1  PzLowerLimitBoundUnits=m  PzLowerLimitStiffness=1e6  PzLowerLimitStiffnessUnits=N/m  PzLowerLimitDamping=1e3  PzLowerLimitDampingUnits=N/(m/s)  PzLowerLimitTransitionRegionWidth=1e-4  PzLowerLimitTransitionRegionWidthUnits=m  PzUpperLimitSpecify=off  PzUpperLimitBound=1  PzUpperLimitBoundUnits=m  PzUpperLimitStiffness=1e6  PzUpperLimitStiffnessUnits=N/m  PzUpperLimitDamping=1e3  PzUpperLimitDampingUnits=N/(m/s)  PzUpperLimitTransitionRegionWidth=1e-4  PzUpperLimitTransitionRegionWidthUnits=m  PzTorqueActuationMode=ComputedTorque  PzMotionActuationMode=InputMotion  PzSensePosition=off  PzSenseVelocity=off  PzSenseAcceleration=off  PzSenseTorqueForce=off  PzSenseLowerLimitTorqueForce=off  PzSenseUpperLimitTorqueForce=off
  Constant : Constant  Value=0
  Origin&Env : Subsystem
  Simulink-PS Converter : nesl_utility/Simulink-PS Converter  PhysicalDomain=network_engine_domain  SubClassName=ps_input  LeftPortType=input  RightPortType=output  PseudoPeriodic=off  Frequencies=[]  NoiseDistribution=none  NoiseParameters=[]  Unit=1  AffineConversion=off  FilteringAndDerivatives=filter  SimscapeFilterOrder=2  InputFilterTimeConstant=0.001  UdotUserProvided=0
  Simulink-PS Converter1 : nesl_utility/Simulink-PS Converter  PhysicalDomain=network_engine_domain  SubClassName=ps_input  LeftPortType=input  RightPortType=output  PseudoPeriodic=off  Frequencies=[]  NoiseDistribution=none  NoiseParameters=[]  Unit=1  AffineConversion=off  FilteringAndDerivatives=filter  SimscapeFilterOrder=2  InputFilterTimeConstant=0.001  UdotUserProvided=0
  Simulink-PS Converter2 : nesl_utility/Simulink-PS Converter  PhysicalDomain=network_engine_domain  SubClassName=ps_input  LeftPortType=input  RightPortType=output  PseudoPeriodic=off  Frequencies=[]  NoiseDistribution=none  NoiseParameters=[]  Unit=1  AffineConversion=off  FilteringAndDerivatives=filter  SimscapeFilterOrder=2  InputFilterTimeConstant=0.001  UdotUserProvided=0
  Spherical Solid : sm_lib/Body Elements/Spherical Solid  SphereRadius=0.1  SphereRadiusUnits=m  ExportEntireGeometry=off  InertiaType=CalculateFromGeometry  BasedOnType=Density  Density=1000  DensityUnits=kg/m^3  Mass=1  MassUnits=kg  CenterOfMass=[0 0 0]  CenterOfMassUnits=m  MomentsOfInertia=[1 1 1]  MomentsOfInertiaUnits=kg*m^2  ProductsOfInertia=[0 0 0]  ProductsOfInertiaUnits=kg*m^2  GraphicType=FromGeometry  MarkerShape=Sphere  MarkerSize=10  GraphicVisPropType=SimpleVisualProperties  GraphicDiffuseColor=[1.0 0.2 0.2]  GraphicOpacity=1.0  GraphicSpecularColor=[0.5 0.5 0.5 1.0]  GraphicAmbientColor=[0.15 0.15 0.15 1.0]  GraphicEmissiveColor=[0.0 0.0 0.0 1.0]  GraphicShininess=75  DoExposeReferenceFrame=on  SerializedFrames=<Frames/>
  wires:
  pz/1 -> Simulink-PS Converter1/1
  px/1 -> Simulink-PS Converter/1
  Constant/1 -> Simulink-PS Converter2/1
  connections:
  Simulink-PS Converter2/RConn1 -- Cartesian Joint/LConn4
  Spherical Solid/RConn1 -- Cartesian Joint/RConn1
  Simulink-PS Converter/RConn1 -- Cartesian Joint/LConn2
  Cartesian Joint/LConn1 -- Origin&Env/LConn1
  Simulink-PS Converter1/RConn1 -- Cartesian Joint/LConn3

== system VirtualMotoTemplate/Rider Commands/Rider Commands/Roll angle control/Rider Steering Control/Rider Steering/Target trajectory driving - Look ahead point/feedback ==
  note: derive target roll angle
  mindist : Inport
  roll : Inport  Port=2
  rollRate : Inport  Port=3
  Gain1 : Gain  Gain=RidTrajContG
  KphiRM : Gain  Gain=RidTrajContGphi
  KphidRM : Gain  Gain=RidTrajContGphid
  Sum : Sum  Inputs=|+-
  Sum1 : Sum  Inputs=|++
  control torque : Outport  VectorParamsAs1DForOutWhenUnconnected=off
  wires:
  roll/1 -> Sum/2
  Gain1/1 -> Sum/1
  rollRate/1 -> KphidRM/1
  KphiRM/1 -> Sum1/1
  KphidRM/1 -> Sum1/2
  Sum/1 -> KphiRM/1
  mindist/1 -> Gain1/1  "mindist"
  Sum1/1 -> control torque/1

== system VirtualMotoTemplate/Rider Commands/Rider Commands/Roll angle control/Rider Steering Control/Rider Steering/Target trajectory driving - Look ahead point/LAPview/Origin&Env ==
  Ground : Subsystem
  Mechanism Configuration : sm_lib/Utilities/Mechanism Configuration  UniformGravity=Constant  GravityVector=[0 0 0]  GravityVectorUnits=m/s^2  LinearizationDelta=0.001  JointModeTransitionNonlinearIterations=2
  Solver Configuration : nesl_utility/Solver Configuration  PhysicalDomain=network_engine_domain  SubClassName=solver  LeftPortType=input  RightPortType=generic  Tones=[]  Harmonics=[]  SimulateNoise=off  Profile=off  UseLocalSampling=off  EnableSwitchedLinearOptims=on  FrequencyDomain=off  UseCCode=off  RelTol=0.001  AbsTol=1e-06  MinStep=1e-09  ToWorkspace=off  RevertToSquareIcSolve=off  NumHomotopyIterations=100  PhasorMode=off  PhasorModeNumHarmonics=1  ConsistencySolver=NEWTON_FTOL  IndexReductionMethod=DerivativeReplacement  DoDC=off  ResidualTolerance=1e-09  ConsistencyTolSource=GLOBAL  ConsistencyAbsTol=0.001  ConsistencyRelTol=0.001  ConsistencyTolFactor=0.001  UseLocalSolver=off  LocalSolverChoice=NE_BACKWARD_EULER_ADVANCER  ResolveIndetEquations=on  FunctionEvalNumThread=1  LocalSolverSampleTime=0.001  DoFixedCost=off  MaxNonlinIter=3  MaxModeIter=2  ComputeImpulses=off  ImpulseIterations=2  LinearAlgebra=Sparse  LinearAlgebraNumThread=0  EquationFormulation=NE_TIME_EF  DelaysMemoryBudget=1024  AutomaticFiltering=on  FilteringTimeConstant=0.001  PartitionStorageMethod=AS_NEEDED  PartitionMemoryBudget=1024  PartitionMethod=FAST  MultibodyUseLocalSolver=off  MultibodyLocalSolverChoice=ODE1  MultibodyLocalSolverSampleTime=0.001
  World Frame : sm_lib/Frames and Transforms/World Frame
  F : PMIOPort  Side=Left
  connections:
  World Frame/RConn1 -- Ground/LConn1 -- F/RConn1 -- Mechanism Configuration/RConn1 -- Solver Configuration/RConn1
